simulink model "BatteryStoragePVPlantGFM"  (R2022b)
settings: Solver=FixedStepDiscrete  StartTime=0.0  StopTime=SimulationTime  RelTol=1e-3
PreLoadFcn:
  | run('BatteryStoragePVPlantGFMParameters')
undefined symbols (not defined in the file): Array, Base, battery, BatteryInverter, DiscIntNeverNeededParam, ee, Feeder, fRT, GFLBatteryController, GFMBatteryController, Grid, GridTransformer, Line, Load, Load2CB_final, Load2CB_initial, LVRT, maxSoC, maxVdc, minIrrad, minSoC, minVdc, Mpp, olTime, Panel, PVController, PVInverter, PVTransformer, Scenario, SM, SubTransmissionLine, Ts, VSMbase
libraries: ee_lib x51, nesl_utility x45, fl_lib x26, eeGeneralControl x18, simulink x12, eeTransforms x11, slpidlib x8, eePowerMeasurement x5, batteryecm_lib x2, eeTotalHarmonicDistorsion x2, spsLeadLagFilterLib x1, eeSmAC1C x1
(part 3 of 5)

== system BatteryStoragePVPlantGFM/BESS & PV PARK/PV Plant Controller /Voltage VAR Control & LVRT, FRT/Voltage Control ==
  In1 : Inport
  In2 : Inport  Port=2
  Constant2 : Constant  Value=0
  Gain : Gain  Gain=PVController.m_v
  Sum2 : Sum  Inputs=|+-
  Switch1 : Switch  Threshold=.9  SaturateOnIntegerOverflow=off  InputSameDT=off
  Out1 : Outport
  wires:
  Gain/1 -> Out1/1
  Sum2/1 -> Switch1/1
  Switch1/1 -> Gain/1
  In1/1 -> Sum2/2, Switch1/2
  Constant2/1 -> Switch1/3
  In2/1 -> Sum2/1

== system BatteryStoragePVPlantGFM/Conventional Source/Variant Subsystem/Frequency Controlled Source/Frequency Control ==
  Pref : Inport
  In Bus Element : Inport  Port=2  PortName=Grid  Element=Pe
  Discrete-Time Integrator : DiscreteIntegrator  IntegratorMethod=Integration: Backward Euler  InitialCondition=0.998  SampleTime=Ts  LimitOutput=on  UpperSaturationLimit=1.1  LowerSaturationLimit=0.9  ICPrevOutput=DiscIntNeverNeededParam  ICPrevScaledInput=DiscIntNeverNeededParam
  Gain2 : Gain  Gain=Grid.frequency
  Gain3 : Gain  Gain=1/Grid.H
  Gain4 : Gain  Gain=Grid.damping*2*pi*Grid.frequency
  Gain6 : Gain  Gain=1/Grid.governor_droop
  Sum : Sum  Inputs=|+-
  Sum1 : Sum  Inputs=-+-|
  Sum2 : Sum  Inputs=|+-
  Sum3 : Sum  Inputs=++|
  Unit Delay : UnitDelay  InitialCondition=1  SampleTime=Grid.sensor_time  HasFrameUpgradeWarning=on
  Unit Delay1 : UnitDelay  InitialCondition=1  SampleTime=Grid.sensor_time  HasFrameUpgradeWarning=on
  w_ref : Constant
  Frequency : Outport
  wires:
  Sum3/1 -> Sum1/2
  w_ref/1 -> Sum2/2, Sum/1
  Sum1/1 -> Gain3/1
  Gain3/1 -> Discrete-Time Integrator/1
  Gain6/1 -> Sum3/2
  Gain2/1 -> Frequency/1
  Sum2/1 -> Gain4/1
  Sum/1 -> Gain6/1
  Pref/1 -> Sum3/1
  Gain4/1 -> Sum1/3
  In Bus Element/1 -> Sum1/1
  Discrete-Time Integrator/1 -> Unit Delay1/1, Unit Delay/1, Gain2/1
  Unit Delay/1 -> Sum/2
  Unit Delay1/1 -> Sum2/1

== system BatteryStoragePVPlantGFM/Conventional Source/Variant Subsystem/Synchronous Machine/AVR and Exciter ==
  Constant{3,5..9} (6 alike) : Constant  Value=0
  Constant4 : Constant
  "E_FD Simulink-PS " : nesl_utility/Simulink-PS Converter  PhysicalDomain=network_engine_domain  SubClassName=ps_input  LeftPortType=input  RightPortType=output  PseudoPeriodic=off  Frequencies=[]  NoiseDistribution=none  NoiseParameters=[]  Unit=1  AffineConversion=off  FilteringAndDerivatives=provide  SimscapeFilterOrder=1  InputFilterTimeConstant=.001  UdotUserProvided=0
  I_FD PS-Simulink : nesl_utility/PS-Simulink Converter  PhysicalDomain=network_engine_domain  SubClassName=ps_output  LeftPortType=input  RightPortType=output  PseudoPeriodic=off  Frequencies=[]  VectorFormat=1-D array  Unit=1  AffineConversion=off
  SM AC1C : eeSmAC1C/SM AC1C  E_FD0=1  Ts=-1  R_C=0  X_C=0  T_R=0  K_A=600  T_A=0.01  T_B=0  T_C=0  K_F=0.35  T_F=0.5  V_Amax=14.5  V_Amin=-14.5  E_FEmax=6.03  E_FEmin=-5.43  oelInputLocation=Unused  uelInputLocation=Unused  sclInputLocation=Unused  K_E=1  T_E=0.08  K_C=0.2  K_D=0.38  E_1=4.18  S_E_E1=0.1  E_2=3.14  S_E_E2=0.03  V_FEmax=99  V_Emin=0
  Synchronous Machine Field Circuit (pu) : ee_lib/Electromechanical/Synchronous/Synchronous Machine Field Circuit  unit_option=ee.enum.unit.pu  SRated=SM.MVA V*A  FRated=60 Hz  fieldCircuitParameterization_option=2  baseEfd=92.95 V  baseIfd=1300 A  parameterization_option=2  Ladu=1.66  Rfd=0.0006  Xl=SM.lekage_reactance  Xd=SM.xd  Xdd=SM.xd_  Xddd=SM.xd_dash  d_option=ee.enum.circuit.open  Td0d=SM.Tdo_ s  Tdd=1.3260 s  Td0dd=SM.Tdo_dash s  Tddd=0.0230 s
      settings: InternalSimscapePortConfiguration="{\"Bottom\":[],\"Left\":[{\"id\":\"Efd_pu\",\"label\":\"Efd_pu\",\"type\":\"input\"},{\"id\":\"Ifd_pu\",\"label\":\"Ifd_pu\",\"type\":\"output\"}],\"Right\":[{\"id\":\"fd_p\",\"label\":\"fd+\",\"type\":\"foundation.electrical.electrical\"},{\"id\":\"fd_n\",\"label\":\"fd-\",\"type\":\"foundation.electrical.electrical\"}],\"Top\":[]}"
  Terminal Current Measurement : ee_lib/Electromechanical/Synchronous/Synchronous Machine Measurement  output_idx=15
      settings: InternalSimscapePortConfiguration="{\"Bottom\":[],\"Left\":[{\"id\":\"pu_input\",\"label\":\"pu\",\"type\":\"input\"}],\"Right\":[{\"id\":\"pu_output\",\"label\":\"o\",\"type\":\"output\"}],\"Top\":[]}"
  Terminal Current PS-Simulink : nesl_utility/PS-Simulink Converter  PhysicalDomain=network_engine_domain  SubClassName=ps_output  LeftPortType=input  RightPortType=output  PseudoPeriodic=off  Frequencies=[]  VectorFormat=1-D array  Unit=1  AffineConversion=off
  Terminal Voltage Measurement : ee_lib/Electromechanical/Synchronous/Synchronous Machine Measurement  output_idx=14
      settings: InternalSimscapePortConfiguration="{\"Bottom\":[],\"Left\":[{\"id\":\"pu_input\",\"label\":\"pu\",\"type\":\"input\"}],\"Right\":[{\"id\":\"pu_output\",\"label\":\"o\",\"type\":\"output\"}],\"Top\":[]}"
  Terminal Voltage PS-Simulink : nesl_utility/PS-Simulink Converter  PhysicalDomain=network_engine_domain  SubClassName=ps_output  LeftPortType=input  RightPortType=output  PseudoPeriodic=off  Frequencies=[]  VectorFormat=1-D array  Unit=1  AffineConversion=off
  Unit Delay : UnitDelay  InitialCondition=1.32943  SampleTime=-1  HasFrameUpgradeWarning=on
  pu : PMIOPort  Side=Left
  fd+ : PMIOPort  Port=2  Side=Right
  fd- : PMIOPort  Port=3  Side=Right
  wires:
  Terminal Current PS-Simulink/1 -> SM AC1C/4
  SM AC1C/1 -> "E_FD Simulink-PS "/1
  Unit Delay/1 -> SM AC1C/10
  Constant9/1 -> SM AC1C/9
  Constant8/1 -> SM AC1C/8
  Constant7/1 -> SM AC1C/7
  Constant6/1 -> SM AC1C/6
  Constant5/1 -> SM AC1C/5
  Constant4/1 -> SM AC1C/1
  Constant3/1 -> SM AC1C/2
  Terminal Voltage PS-Simulink/1 -> SM AC1C/3
  I_FD PS-Simulink/1 -> Unit Delay/1
  connections:
  Terminal Current Measurement/RConn1 -- Terminal Current PS-Simulink/LConn1
  Terminal Voltage Measurement/RConn1 -- Terminal Voltage PS-Simulink/LConn1
  pu/RConn1 -- Terminal Current Measurement/LConn1 -- Terminal Voltage Measurement/LConn1
  Synchronous Machine Field Circuit (pu)/RConn1 -- fd+/RConn1
  fd-/RConn1 -- Synchronous Machine Field Circuit (pu)/RConn2
  I_FD PS-Simulink/LConn1 -- Synchronous Machine Field Circuit (pu)/LConn2
  "E_FD Simulink-PS "/RConn1 -- Synchronous Machine Field Circuit (pu)/LConn1

== system BatteryStoragePVPlantGFM/Conventional Source/Variant Subsystem/Synchronous Machine/CB4 ==
  Circuit Breaker Step off3 : ee_lib/Switches & Breakers/Circuit Breaker (Three-Phase)  R_closed=0.001 Ohm  G_open=1e-4 1/Ohm  threshold=0.5 V  breaker_behavior=ee.enum.switches.breakerBehavior.zeroCrossingEnable
      settings: InternalSimscapePortConfiguration="{\"Bottom\":[],\"Left\":[{\"id\":\"vT\",\"label\":\"vT\",\"type\":\"input\"},{\"id\":\"N1\",\"label\":\"~1\",\"type\":\"foundation.electrical.three_phase\"}],\"Right\":[{\"id\":\"N2\",\"label\":\"~2\",\"type\":\"foundation.electrical.three_phase\"}],\"Top\":[]}"
  Simulink-PS Converter3 : nesl_utility/Simulink-PS Converter  PhysicalDomain=network_engine_domain  SubClassName=ps_input  LeftPortType=input  RightPortType=output  PseudoPeriodic=off  Frequencies=[]  NoiseDistribution=none  NoiseParameters=[]  Unit=1  AffineConversion=off  FilteringAndDerivatives=zero  SimscapeFilterOrder=1  InputFilterTimeConstant=0.001  UdotUserProvided=1
  Step off3 : Step  Time=0  After=0  SampleTime=Ts
  Conn2 : PMIOPort  Side=Left
  Conn1 : PMIOPort  Port=2  Side=Right
  wires:
  Step off3/1 -> Simulink-PS Converter3/1
  connections:
  Circuit Breaker Step off3/LConn2 -- Conn2/RConn1
  Circuit Breaker Step off3/LConn1 -- Simulink-PS Converter3/RConn1
  Circuit Breaker Step off3/RConn1 -- Conn1/RConn1

== system BatteryStoragePVPlantGFM/Conventional Source/Variant Subsystem/Synchronous Machine/Governor and Prime Mover  ==
  Governor : Subsystem
  Ideal Torque Source : fl_lib/Mechanical/Mechanical Sources/Ideal Torque Source
  Mechanical Rotational Reference : fl_lib/Mechanical/Rotational Elements/Mechanical Rotational Reference
  Non-reheat turbine : Subsystem
  PS-Simulink Converter : nesl_utility/PS-Simulink Converter  PhysicalDomain=network_engine_domain  SubClassName=ps_output  LeftPortType=input  RightPortType=output  PseudoPeriodic=off  Frequencies=[]  VectorFormat=1-D array  Unit=1  AffineConversion=off
  Rotor Velocity Measurement : ee_lib/Electromechanical/Synchronous/Synchronous Machine Measurement  output_idx=4
      settings: InternalSimscapePortConfiguration="{\"Bottom\":[],\"Left\":[{\"id\":\"pu_input\",\"label\":\"pu\",\"type\":\"input\"}],\"Right\":[{\"id\":\"pu_output\",\"label\":\"o\",\"type\":\"output\"}],\"Top\":[]}"
  Simulink-PS Converter : nesl_utility/Simulink-PS Converter  PhysicalDomain=network_engine_domain  SubClassName=ps_input  LeftPortType=input  RightPortType=output  PseudoPeriodic=off  Frequencies=[]  NoiseDistribution=none  NoiseParameters=[]  Unit=1  AffineConversion=off  FilteringAndDerivatives=zero  SimscapeFilterOrder=1  InputFilterTimeConstant=0.001  UdotUserProvided=1
  scale by base_torque : Gain  Gain=base_torque
  R : PMIOPort  Side=Right
  C : PMIOPort  Port=2  Side=Right
  pu : PMIOPort  Port=3  Side=Left
  wires:
  PS-Simulink Converter/1 -> Governor/1(pu_velocity)
  Governor/1(delta_y) -> Non-reheat turbine/1(delta_y)
  Non-reheat turbine/1(torque) -> scale by base_torque/1
  scale by base_torque/1 -> Simulink-PS Converter/1
  connections:
  C/RConn1 -- Ideal Torque Source/RConn2 -- Mechanical Rotational Reference/LConn1
  Ideal Torque Source/LConn1 -- R/RConn1
  pu/RConn1 -- Rotor Velocity Measurement/LConn1
  PS-Simulink Converter/LConn1 -- Rotor Velocity Measurement/RConn1
  Simulink-PS Converter/RConn1 -- Ideal Torque Source/RConn1

== system BatteryStoragePVPlantGFM/BESS & PV PARK/100 MWp PV Park/PV Inverter A1/PV & Inverter/Measurement1 ==
  u : Inport
  Lead-Lag (Discrete or Continuous) : eeGeneralControl/Lead-Lag (Discrete or Continuous)  T1=0  T2=PVController.t_sensor  B=inf  A=-inf  init_option=Inherited from block input  x0=0  Ts=Ts
      settings: LibrarySourceBlock=|
      | ee_sl_lib/General Control/Lead-Lag
      | (Discrete or Continuous)
  Out1 : Outport
  wires:
  Lead-Lag (Discrete or Continuous)/1 -> Out1/1
  u/1 -> Lead-Lag (Discrete or Continuous)/1

== system BatteryStoragePVPlantGFM/BESS & PV PARK/100 MWp PV Park/PV Inverter A1/PV & Inverter/Measurement2 ==
  u : Inport
  Lead-Lag (Discrete or Continuous) : eeGeneralControl/Lead-Lag (Discrete or Continuous)  T1=0  T2=PVController.t_sensor  B=inf  A=-inf  init_option=Inherited from block input  x0=0  Ts=Ts
      settings: LibrarySourceBlock=|
      | ee_sl_lib/General Control/Lead-Lag
      | (Discrete or Continuous)
  Out1 : Outport
  wires:
  Lead-Lag (Discrete or Continuous)/1 -> Out1/1
  u/1 -> Lead-Lag (Discrete or Continuous)/1

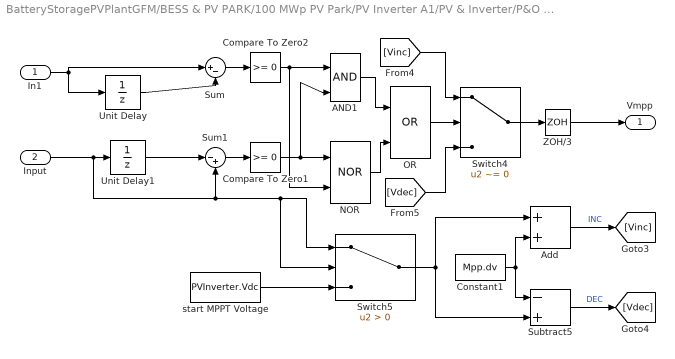
== system BatteryStoragePVPlantGFM/BESS & PV PARK/100 MWp PV Park/PV Inverter A1/PV & Inverter/P&O MPP ==
  In1 : Inport
  Input : Inport  Port=2
  AND1 : Logic  IconShape=distinctive  AllPortsSameDT=off  OutDataTypeStr=boolean
  Add : Sum
  Compare To Zero1 : simulink/Logic and Bit Operations/Compare To Zero  relop=>=  OutDataTypeStr=boolean
  Compare To Zero2 : simulink/Logic and Bit Operations/Compare To Zero  relop=>=  OutDataTypeStr=boolean
  Constant1 : Constant  Value=Mpp.dv
  NOR : Logic  Operator=NOR  IconShape=distinctive  AllPortsSameDT=off  OutDataTypeStr=boolean
  OR : Logic  Operator=OR  IconShape=distinctive  AllPortsSameDT=off  OutDataTypeStr=boolean
  Subtract5 : Sum  Inputs=-+
  Sum : Sum  Inputs=|+-
  Sum1 : Sum  Inputs=|-+
  Switch4 : Switch  Criteria=u2 ~= 0  SaturateOnIntegerOverflow=off  InputSameDT=off
  Switch5 : Switch  Criteria=u2 > Threshold  SaturateOnIntegerOverflow=off  InputSameDT=off
  Unit Delay : UnitDelay  InitialCondition=2.5e5  SampleTime=Mpp.ts  HasFrameUpgradeWarning=on
  Unit Delay1 : UnitDelay  InitialCondition=1*PVInverter.Vdc  SampleTime=Mpp.ts  HasFrameUpgradeWarning=on
  ZOH/3 : ZeroOrderHold  SampleTime=Mpp.td
  start MPPT Voltage : Constant  Value=PVInverter.Vdc  SampleTime=Ts
  Vmpp : Outport  VectorParamsAs1DForOutWhenUnconnected=off
  wires:
  OR/1 -> Switch4/2
  Compare To Zero1/1 -> NOR/1, AND1/2
  start MPPT Voltage/1 -> Switch5/3
  Compare To Zero2/1 -> NOR/2, AND1/1
  In1/1 -> Unit Delay/1, Sum/1
  Switch5/1 -> Add/1, Subtract5/2
  Constant1/1 -> Add/2, Subtract5/1
  Input/1 -> Switch5/2, Switch5/1, Sum1/2, Unit Delay1/1
  Unit Delay1/1 -> Sum1/1
  Add/1 -> [Vinc]  "INC"
  NOR/1 -> OR/2
  Subtract5/1 -> [Vdec]  "DEC"
  [Vdec] -> Switch4/3
  Switch4/1 -> ZOH/3/1
  Sum1/1 -> Compare To Zero1/1
  Sum/1 -> Compare To Zero2/1
  AND1/1 -> OR/1
  Unit Delay/1 -> Sum/2
  ZOH/3/1 -> Vmpp/1
  [Vinc] -> Switch4/1

== system BatteryStoragePVPlantGFM/BESS & PV PARK/100 MWp PV Park/PV Inverter A1/PV Controller/Current_controller ==
  id-ref : Inport
  ipvd : Inport  Port=2
  iqref : Inport  Port=3
  iq : Inport  Port=4
  Vd : Inport  Port=5
  Vq : Inport  Port=6
  Constant4 : Constant  Value=0
  Gain1 : Gain  Gain=2*1*pi*60*PVInverter.L/Base.z_base
  Gain2 : Gain  Gain=2*1*pi*60*PVInverter.L/Base.z_base
  Mux1 : Mux  Inputs=3
  PID Controller : slpidlib/PID Controller  Controller=PID  Form=Parallel  TimeDomain=Discrete-time  UseExternalTs=off  SampleTime=-1  IntegratorMethod=Forward Euler  FilterMethod=Forward Euler  ControllerParametersSource=internal  P=PVController.Kp_ic  I=PVController.Ki_ic  UseKiTs=off  D=PVController.Kd  N=100  UseFilter=on  TunerSelectOption=Transfer Function Based (PID Tuner App)  InitialConditionSource=internal  InitialConditionForIntegrator=0  InitialConditionForFilter=0  DifferentiatorICPrevScaledInput=0  ExternalReset=none  TrackingMode=off  Kt=1  LimitOutput=off  SatLimitsSource=internal  UpperSaturationLimit=inf  LowerSaturationLimit=-inf  LinearizeAsGain=on  AntiWindupMode=none  Kb=1  LimitIntegrator=off  UpperIntegratorSaturationLimit=inf  LowerIntegratorSaturationLimit=-inf  POutMin=[]  POutMax=[]  IOutMin=[]  IOutMax=[]  DOutMin=[]  DOutMax=[]  NOutMin=[]  NOutMax=[]  SumOutMin=[]  SumOutMax=[]  SaturationOutMin=[]  SaturationOutMax=[]  PParamMin=[]  PParamMax=[]  IParamMin=[]  IParamMax=[]  DParamMin=[]  DParamMax=[]  NParamMin=[]  NParamMax=[]  KbParamMin=[]  KbParamMax=[]  KtParamMin=[]  KtParamMax=[]  KbOutMin=[]  KbOutMax=[]  KtOutMin=[]  KtOutMax=[]  IntegratorOutMin=[]  IntegratorOutMax=[]  FilterOutMin=[]  FilterOutMax=[]  SumI1OutMin=[]  SumI1OutMax=[]  SumI2OutMin=[]  SumI2OutMax=[]  SumI3OutMin=[]  SumI3OutMax=[]  SumI4OutMin=[]  SumI4OutMax=[]  SumDOutMin=[]  SumDOutMax=[]  DifferentiatorOutMin=[]  DifferentiatorOutMax=[]  FilterDiffOutCoefMin=[]  FilterDiffOutCoefMax=[]  ReciprocalOutMin=[]  ReciprocalOutMax=[]  SumDenOutMin=[]  SumDenOutMax=[]  SumNumOutMin=[]  SumNumOutMax=[]  DivideOutMin=[]  DivideOutMax=[]  UdiffTsProdOutMin=[]  UdiffTsProdOutMax=[]  NTsProdOutMin=[]  NTsProdOutMax=[]  UintegralTsProdOutMin=[]  UintegralTsProdOutMax=[]  UngainTsProdOutMin=[]  UngainTsProdOutMax=[]  ClampingZeroOutDataTypeStr=Inherit: Inherit via back propagation  ClampingZeroOutMin=[]  ClampingZeroOutMax=[]  FilterDenConstantOutDataTypeStr=Inherit: Inherit via back propagation  FilterDenConstantOutMin=[]  FilterDenConstantOutMax=[]  PCopyOutDataTypeStr=Inherit: Inherit via back propagation  PCopyOutMin=[]  PCopyOutMax=[]  NCopyOutDataTypeStr=Inherit: Inherit via back propagation  NCopyOutMin=[]  NCopyOutMax=[]  IntegratorContinuousStateAttributes=''  IntegratorStateMustResolveToSignalObject=off  IntegratorRTWStateStorageClass=Auto  FilterContinuousStateAttributes=''  FilterStateMustResolveToSignalObject=off  FilterRTWStateStorageClass=Auto  ParallelPVariant=InternalParameters  IdealPVariant=Disabled  IVariant=InternalParameters  DVariant=InternalParameters  IntegratorVariant=Discrete  SatVariant=Disabled  AWVariant=Passthrough  PCopyVariant=Disabled  TRVariant=Disabled  FdbkBlocksVariant=Forward  IdealPFdbkVariant=Disabled  SatFdbkVariant=Disabled  DerivativeFilterVariant=ForwardEulerFilter  NVariant=InternalParameters  NCopyVariant=Disabled  FilterICVariant=InternalICsFilter  IntegratorICVariant=InternalICs  ExternalResetVariant=Disabled  TRSumVariant=Passthrough  SumFdbkVariant=Disabled  SumVariant=Sum_PID  TsampFilterVariant=InternalTs  TsampNgainVariant=Passthrough  TsampIntegralVariant=Passthrough  ExternalSaturationOutDataTypeStr=Inherit: Same as second input
  PID Controller1 : slpidlib/PID Controller  Controller=PID  Form=Parallel  TimeDomain=Discrete-time  UseExternalTs=off  SampleTime=-1  IntegratorMethod=Forward Euler  FilterMethod=Forward Euler  ControllerParametersSource=internal  P=PVController.Kp_ic  I=PVController.Ki_ic  UseKiTs=off  D=PVController.Kd  N=100  UseFilter=on  TunerSelectOption=Transfer Function Based (PID Tuner App)  InitialConditionSource=internal  InitialConditionForIntegrator=0  InitialConditionForFilter=0  DifferentiatorICPrevScaledInput=0  ExternalReset=none  TrackingMode=off  Kt=1  LimitOutput=off  SatLimitsSource=internal  UpperSaturationLimit=inf  LowerSaturationLimit=-inf  LinearizeAsGain=on  AntiWindupMode=none  Kb=1  LimitIntegrator=off  UpperIntegratorSaturationLimit=inf  LowerIntegratorSaturationLimit=-inf  POutMin=[]  POutMax=[]  IOutMin=[]  IOutMax=[]  DOutMin=[]  DOutMax=[]  NOutMin=[]  NOutMax=[]  SumOutMin=[]  SumOutMax=[]  SaturationOutMin=[]  SaturationOutMax=[]  PParamMin=[]  PParamMax=[]  IParamMin=[]  IParamMax=[]  DParamMin=[]  DParamMax=[]  NParamMin=[]  NParamMax=[]  KbParamMin=[]  KbParamMax=[]  KtParamMin=[]  KtParamMax=[]  KbOutMin=[]  KbOutMax=[]  KtOutMin=[]  KtOutMax=[]  IntegratorOutMin=[]  IntegratorOutMax=[]  FilterOutMin=[]  FilterOutMax=[]  SumI1OutMin=[]  SumI1OutMax=[]  SumI2OutMin=[]  SumI2OutMax=[]  SumI3OutMin=[]  SumI3OutMax=[]  SumI4OutMin=[]  SumI4OutMax=[]  SumDOutMin=[]  SumDOutMax=[]  DifferentiatorOutMin=[]  DifferentiatorOutMax=[]  FilterDiffOutCoefMin=[]  FilterDiffOutCoefMax=[]  ReciprocalOutMin=[]  ReciprocalOutMax=[]  SumDenOutMin=[]  SumDenOutMax=[]  SumNumOutMin=[]  SumNumOutMax=[]  DivideOutMin=[]  DivideOutMax=[]  UdiffTsProdOutMin=[]  UdiffTsProdOutMax=[]  NTsProdOutMin=[]  NTsProdOutMax=[]  UintegralTsProdOutMin=[]  UintegralTsProdOutMax=[]  UngainTsProdOutMin=[]  UngainTsProdOutMax=[]  ClampingZeroOutDataTypeStr=Inherit: Inherit via back propagation  ClampingZeroOutMin=[]  ClampingZeroOutMax=[]  FilterDenConstantOutDataTypeStr=Inherit: Inherit via back propagation  FilterDenConstantOutMin=[]  FilterDenConstantOutMax=[]  PCopyOutDataTypeStr=Inherit: Inherit via back propagation  PCopyOutMin=[]  PCopyOutMax=[]  NCopyOutDataTypeStr=Inherit: Inherit via back propagation  NCopyOutMin=[]  NCopyOutMax=[]  IntegratorContinuousStateAttributes=''  IntegratorStateMustResolveToSignalObject=off  IntegratorRTWStateStorageClass=Auto  FilterContinuousStateAttributes=''  FilterStateMustResolveToSignalObject=off  FilterRTWStateStorageClass=Auto  ParallelPVariant=InternalParameters  IdealPVariant=Disabled  IVariant=InternalParameters  DVariant=InternalParameters  IntegratorVariant=Discrete  SatVariant=Disabled  AWVariant=Passthrough  PCopyVariant=Disabled  TRVariant=Disabled  FdbkBlocksVariant=Forward  IdealPFdbkVariant=Disabled  SatFdbkVariant=Disabled  DerivativeFilterVariant=ForwardEulerFilter  NVariant=InternalParameters  NCopyVariant=Disabled  FilterICVariant=InternalICsFilter  IntegratorICVariant=InternalICs  ExternalResetVariant=Disabled  TRSumVariant=Passthrough  SumFdbkVariant=Disabled  SumVariant=Sum_PID  TsampFilterVariant=InternalTs  TsampNgainVariant=Passthrough  TsampIntegralVariant=Passthrough  ExternalSaturationOutDataTypeStr=Inherit: Same as second input
  Sum1 : Sum  Inputs=|+-
  Sum3 : Sum  Inputs=|++-
  Sum4 : Sum  Inputs=|+++
  Sum5 : Sum  Inputs=|+-
  Refrence_mdq0 : Outport
  wires:
  PID Controller/1 -> Sum3/2
  Sum3/1 -> Mux1/1, [Ed]
  Gain2/1 -> Sum3/3
  ipvd/1 -> Gain1/1, Sum1/2
  id-ref/1 -> Sum1/1
  Gain1/1 -> Sum4/3
  Vq/1 -> Sum4/2
  iq/1 -> Gain2/1, Sum5/2
  Sum1/1 -> PID Controller/1
  Vd/1 -> Sum3/1
  Constant4/1 -> Mux1/3
  Sum5/1 -> PID Controller1/1
  iqref/1 -> Sum5/1
  PID Controller1/1 -> Sum4/1
  Sum4/1 -> Mux1/2, [Eq]
  Mux1/1 -> Refrence_mdq0/1  "m_dqo"

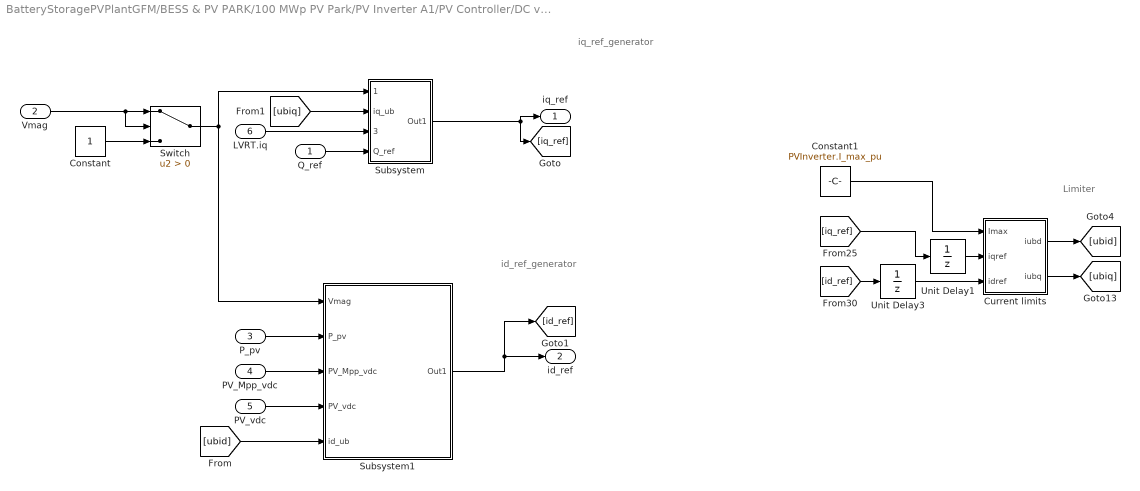
== system BatteryStoragePVPlantGFM/BESS & PV PARK/100 MWp PV Park/PV Inverter A1/PV Controller/DC voltage controller & current reference ==
  note: Limiter
  note: iq_ref_generator
  note: id_ref_generator
  Q_ref : Inport
  Vmag : Inport  Port=2
  P_pv : Inport  Port=3
  PV_Mpp_vdc : Inport  Port=4
  PV_vdc : Inport  Port=5
  LVRT.iq : Inport  Port=6
  Constant : Constant
  Constant1 : Constant  Value=PVInverter.I_max_pu
  Current limits : Subsystem
  Subsystem : Subsystem
  Subsystem1 : Subsystem
  Switch : Switch  Criteria=u2 > Threshold  SaturateOnIntegerOverflow=off  InputSameDT=off
  Unit Delay1 : UnitDelay  SampleTime=Ts  HasFrameUpgradeWarning=on
  Unit Delay3 : UnitDelay  SampleTime=Ts  HasFrameUpgradeWarning=on
  iq_ref : Outport
  id_ref : Outport  Port=2
  wires:
  Vmag/1 -> Switch/2, Switch/1
  [iq_ref] -> Unit Delay1/1
  Current limits/2(iubq) -> [ubiq]
  Current limits/1(iubd) -> [ubid]
  Constant1/1 -> Current limits/1(Imax)
  Unit Delay1/1 -> Current limits/2(iqref)
  [id_ref] -> Unit Delay3/1
  Unit Delay3/1 -> Current limits/3(idref)
  Q_ref/1 -> Subsystem/4(Q_ref)
  Subsystem1/1(Out1) -> [id_ref], id_ref/1
  P_pv/1 -> Subsystem1/2(P_pv)
  PV_Mpp_vdc/1 -> Subsystem1/3(PV_Mpp_vdc)
  PV_vdc/1 -> Subsystem1/4(PV_vdc)
  Subsystem/1(Out1) -> [iq_ref], iq_ref/1
  [ubid] -> Subsystem1/5(id_ub)
  [ubiq] -> Subsystem/2(iq_ub)
  LVRT.iq/1 -> Subsystem/3(LVRT.iq)
  Switch/1 -> Subsystem/1(V_mag), Subsystem1/1(Vmag)
  Constant/1 -> Switch/3

== system BatteryStoragePVPlantGFM/BESS & PV PARK/100 MWp PV Park/PV Inverter A2/PV & Inverter/Measurement1 ==
  u : Inport
  Lead-Lag (Discrete or Continuous) : eeGeneralControl/Lead-Lag (Discrete or Continuous)  T1=0  T2=PVController.t_sensor  B=inf  A=-inf  init_option=Inherited from block input  x0=0  Ts=Ts
      settings: LibrarySourceBlock=|
      | ee_sl_lib/General Control/Lead-Lag
      | (Discrete or Continuous)
  Out1 : Outport
  wires:
  Lead-Lag (Discrete or Continuous)/1 -> Out1/1
  u/1 -> Lead-Lag (Discrete or Continuous)/1

== system BatteryStoragePVPlantGFM/BESS & PV PARK/100 MWp PV Park/PV Inverter A2/PV & Inverter/Measurement2 ==
  u : Inport
  Lead-Lag (Discrete or Continuous) : eeGeneralControl/Lead-Lag (Discrete or Continuous)  T1=0  T2=PVController.t_sensor  B=inf  A=-inf  init_option=Inherited from block input  x0=0  Ts=Ts
      settings: LibrarySourceBlock=|
      | ee_sl_lib/General Control/Lead-Lag
      | (Discrete or Continuous)
  Out1 : Outport
  wires:
  Lead-Lag (Discrete or Continuous)/1 -> Out1/1
  u/1 -> Lead-Lag (Discrete or Continuous)/1

== system BatteryStoragePVPlantGFM/BESS & PV PARK/100 MWp PV Park/PV Inverter A2/PV & Inverter/P&O MPP ==
  In1 : Inport
  Input : Inport  Port=2
  AND1 : Logic  IconShape=distinctive  AllPortsSameDT=off  OutDataTypeStr=boolean
  Add : Sum
  Compare To Zero1 : simulink/Logic and Bit Operations/Compare To Zero  relop=>=  OutDataTypeStr=boolean
  Compare To Zero2 : simulink/Logic and Bit Operations/Compare To Zero  relop=>=  OutDataTypeStr=boolean
  Constant1 : Constant  Value=Mpp.dv
  NOR : Logic  Operator=NOR  IconShape=distinctive  AllPortsSameDT=off  OutDataTypeStr=boolean
  OR : Logic  Operator=OR  IconShape=distinctive  AllPortsSameDT=off  OutDataTypeStr=boolean
  Subtract5 : Sum  Inputs=-+
  Sum : Sum  Inputs=|+-
  Sum1 : Sum  Inputs=|-+
  Switch4 : Switch  Criteria=u2 ~= 0  SaturateOnIntegerOverflow=off  InputSameDT=off
  Switch5 : Switch  Criteria=u2 > Threshold  SaturateOnIntegerOverflow=off  InputSameDT=off
  Unit Delay : UnitDelay  InitialCondition=2.5e5  SampleTime=Mpp.ts  HasFrameUpgradeWarning=on
  Unit Delay1 : UnitDelay  InitialCondition=1*PVInverter.Vdc  SampleTime=Mpp.ts  HasFrameUpgradeWarning=on
  ZOH/3 : ZeroOrderHold  SampleTime=Mpp.td
  start MPPT Voltage : Constant  Value=PVInverter.Vdc  SampleTime=Ts
  Vmpp : Outport  VectorParamsAs1DForOutWhenUnconnected=off
  wires:
  OR/1 -> Switch4/2
  Compare To Zero1/1 -> NOR/1, AND1/2
  start MPPT Voltage/1 -> Switch5/3
  Compare To Zero2/1 -> NOR/2, AND1/1
  In1/1 -> Unit Delay/1, Sum/1
  Switch5/1 -> Add/1, Subtract5/2
  Constant1/1 -> Add/2, Subtract5/1
  Input/1 -> Switch5/2, Switch5/1, Sum1/2, Unit Delay1/1
  Unit Delay1/1 -> Sum1/1
  Add/1 -> [Vinc]  "INC"
  NOR/1 -> OR/2
  Subtract5/1 -> [Vdec]  "DEC"
  [Vdec] -> Switch4/3
  Switch4/1 -> ZOH/3/1
  Sum1/1 -> Compare To Zero1/1
  Sum/1 -> Compare To Zero2/1
  AND1/1 -> OR/1
  Unit Delay/1 -> Sum/2
  ZOH/3/1 -> Vmpp/1
  [Vinc] -> Switch4/1

== system BatteryStoragePVPlantGFM/BESS & PV PARK/100 MWp PV Park/PV Inverter A2/PV Controller/Current_controller ==
  id-ref : Inport
  ipvd : Inport  Port=2
  iqref : Inport  Port=3
  iq : Inport  Port=4
  Vd : Inport  Port=5
  Vq : Inport  Port=6
  Constant4 : Constant  Value=0
  Gain1 : Gain  Gain=2*1*pi*60*PVInverter.L/Base.z_base
  Gain2 : Gain  Gain=2*1*pi*60*PVInverter.L/Base.z_base
  Mux1 : Mux  Inputs=3
  PID Controller : slpidlib/PID Controller  Controller=PID  Form=Parallel  TimeDomain=Discrete-time  UseExternalTs=off  SampleTime=-1  IntegratorMethod=Forward Euler  FilterMethod=Forward Euler  ControllerParametersSource=internal  P=PVController.Kp_ic  I=PVController.Ki_ic  UseKiTs=off  D=PVController.Kd  N=100  UseFilter=on  TunerSelectOption=Transfer Function Based (PID Tuner App)  InitialConditionSource=internal  InitialConditionForIntegrator=0  InitialConditionForFilter=0  DifferentiatorICPrevScaledInput=0  ExternalReset=none  TrackingMode=off  Kt=1  LimitOutput=off  SatLimitsSource=internal  UpperSaturationLimit=inf  LowerSaturationLimit=-inf  LinearizeAsGain=on  AntiWindupMode=none  Kb=1  LimitIntegrator=off  UpperIntegratorSaturationLimit=inf  LowerIntegratorSaturationLimit=-inf  POutMin=[]  POutMax=[]  IOutMin=[]  IOutMax=[]  DOutMin=[]  DOutMax=[]  NOutMin=[]  NOutMax=[]  SumOutMin=[]  SumOutMax=[]  SaturationOutMin=[]  SaturationOutMax=[]  PParamMin=[]  PParamMax=[]  IParamMin=[]  IParamMax=[]  DParamMin=[]  DParamMax=[]  NParamMin=[]  NParamMax=[]  KbParamMin=[]  KbParamMax=[]  KtParamMin=[]  KtParamMax=[]  KbOutMin=[]  KbOutMax=[]  KtOutMin=[]  KtOutMax=[]  IntegratorOutMin=[]  IntegratorOutMax=[]  FilterOutMin=[]  FilterOutMax=[]  SumI1OutMin=[]  SumI1OutMax=[]  SumI2OutMin=[]  SumI2OutMax=[]  SumI3OutMin=[]  SumI3OutMax=[]  SumI4OutMin=[]  SumI4OutMax=[]  SumDOutMin=[]  SumDOutMax=[]  DifferentiatorOutMin=[]  DifferentiatorOutMax=[]  FilterDiffOutCoefMin=[]  FilterDiffOutCoefMax=[]  ReciprocalOutMin=[]  ReciprocalOutMax=[]  SumDenOutMin=[]  SumDenOutMax=[]  SumNumOutMin=[]  SumNumOutMax=[]  DivideOutMin=[]  DivideOutMax=[]  UdiffTsProdOutMin=[]  UdiffTsProdOutMax=[]  NTsProdOutMin=[]  NTsProdOutMax=[]  UintegralTsProdOutMin=[]  UintegralTsProdOutMax=[]  UngainTsProdOutMin=[]  UngainTsProdOutMax=[]  ClampingZeroOutDataTypeStr=Inherit: Inherit via back propagation  ClampingZeroOutMin=[]  ClampingZeroOutMax=[]  FilterDenConstantOutDataTypeStr=Inherit: Inherit via back propagation  FilterDenConstantOutMin=[]  FilterDenConstantOutMax=[]  PCopyOutDataTypeStr=Inherit: Inherit via back propagation  PCopyOutMin=[]  PCopyOutMax=[]  NCopyOutDataTypeStr=Inherit: Inherit via back propagation  NCopyOutMin=[]  NCopyOutMax=[]  IntegratorContinuousStateAttributes=''  IntegratorStateMustResolveToSignalObject=off  IntegratorRTWStateStorageClass=Auto  FilterContinuousStateAttributes=''  FilterStateMustResolveToSignalObject=off  FilterRTWStateStorageClass=Auto  ParallelPVariant=InternalParameters  IdealPVariant=Disabled  IVariant=InternalParameters  DVariant=InternalParameters  IntegratorVariant=Discrete  SatVariant=Disabled  AWVariant=Passthrough  PCopyVariant=Disabled  TRVariant=Disabled  FdbkBlocksVariant=Forward  IdealPFdbkVariant=Disabled  SatFdbkVariant=Disabled  DerivativeFilterVariant=ForwardEulerFilter  NVariant=InternalParameters  NCopyVariant=Disabled  FilterICVariant=InternalICsFilter  IntegratorICVariant=InternalICs  ExternalResetVariant=Disabled  TRSumVariant=Passthrough  SumFdbkVariant=Disabled  SumVariant=Sum_PID  TsampFilterVariant=InternalTs  TsampNgainVariant=Passthrough  TsampIntegralVariant=Passthrough  ExternalSaturationOutDataTypeStr=Inherit: Same as second input
  PID Controller1 : slpidlib/PID Controller  Controller=PID  Form=Parallel  TimeDomain=Discrete-time  UseExternalTs=off  SampleTime=-1  IntegratorMethod=Forward Euler  FilterMethod=Forward Euler  ControllerParametersSource=internal  P=PVController.Kp_ic  I=PVController.Ki_ic  UseKiTs=off  D=PVController.Kd  N=100  UseFilter=on  TunerSelectOption=Transfer Function Based (PID Tuner App)  InitialConditionSource=internal  InitialConditionForIntegrator=0  InitialConditionForFilter=0  DifferentiatorICPrevScaledInput=0  ExternalReset=none  TrackingMode=off  Kt=1  LimitOutput=off  SatLimitsSource=internal  UpperSaturationLimit=inf  LowerSaturationLimit=-inf  LinearizeAsGain=on  AntiWindupMode=none  Kb=1  LimitIntegrator=off  UpperIntegratorSaturationLimit=inf  LowerIntegratorSaturationLimit=-inf  POutMin=[]  POutMax=[]  IOutMin=[]  IOutMax=[]  DOutMin=[]  DOutMax=[]  NOutMin=[]  NOutMax=[]  SumOutMin=[]  SumOutMax=[]  SaturationOutMin=[]  SaturationOutMax=[]  PParamMin=[]  PParamMax=[]  IParamMin=[]  IParamMax=[]  DParamMin=[]  DParamMax=[]  NParamMin=[]  NParamMax=[]  KbParamMin=[]  KbParamMax=[]  KtParamMin=[]  KtParamMax=[]  KbOutMin=[]  KbOutMax=[]  KtOutMin=[]  KtOutMax=[]  IntegratorOutMin=[]  IntegratorOutMax=[]  FilterOutMin=[]  FilterOutMax=[]  SumI1OutMin=[]  SumI1OutMax=[]  SumI2OutMin=[]  SumI2OutMax=[]  SumI3OutMin=[]  SumI3OutMax=[]  SumI4OutMin=[]  SumI4OutMax=[]  SumDOutMin=[]  SumDOutMax=[]  DifferentiatorOutMin=[]  DifferentiatorOutMax=[]  FilterDiffOutCoefMin=[]  FilterDiffOutCoefMax=[]  ReciprocalOutMin=[]  ReciprocalOutMax=[]  SumDenOutMin=[]  SumDenOutMax=[]  SumNumOutMin=[]  SumNumOutMax=[]  DivideOutMin=[]  DivideOutMax=[]  UdiffTsProdOutMin=[]  UdiffTsProdOutMax=[]  NTsProdOutMin=[]  NTsProdOutMax=[]  UintegralTsProdOutMin=[]  UintegralTsProdOutMax=[]  UngainTsProdOutMin=[]  UngainTsProdOutMax=[]  ClampingZeroOutDataTypeStr=Inherit: Inherit via back propagation  ClampingZeroOutMin=[]  ClampingZeroOutMax=[]  FilterDenConstantOutDataTypeStr=Inherit: Inherit via back propagation  FilterDenConstantOutMin=[]  FilterDenConstantOutMax=[]  PCopyOutDataTypeStr=Inherit: Inherit via back propagation  PCopyOutMin=[]  PCopyOutMax=[]  NCopyOutDataTypeStr=Inherit: Inherit via back propagation  NCopyOutMin=[]  NCopyOutMax=[]  IntegratorContinuousStateAttributes=''  IntegratorStateMustResolveToSignalObject=off  IntegratorRTWStateStorageClass=Auto  FilterContinuousStateAttributes=''  FilterStateMustResolveToSignalObject=off  FilterRTWStateStorageClass=Auto  ParallelPVariant=InternalParameters  IdealPVariant=Disabled  IVariant=InternalParameters  DVariant=InternalParameters  IntegratorVariant=Discrete  SatVariant=Disabled  AWVariant=Passthrough  PCopyVariant=Disabled  TRVariant=Disabled  FdbkBlocksVariant=Forward  IdealPFdbkVariant=Disabled  SatFdbkVariant=Disabled  DerivativeFilterVariant=ForwardEulerFilter  NVariant=InternalParameters  NCopyVariant=Disabled  FilterICVariant=InternalICsFilter  IntegratorICVariant=InternalICs  ExternalResetVariant=Disabled  TRSumVariant=Passthrough  SumFdbkVariant=Disabled  SumVariant=Sum_PID  TsampFilterVariant=InternalTs  TsampNgainVariant=Passthrough  TsampIntegralVariant=Passthrough  ExternalSaturationOutDataTypeStr=Inherit: Same as second input
  Sum1 : Sum  Inputs=|+-
  Sum3 : Sum  Inputs=|++-
  Sum4 : Sum  Inputs=|+++
  Sum5 : Sum  Inputs=|+-
  Refrence_mdq0 : Outport
  wires:
  PID Controller/1 -> Sum3/2
  Sum3/1 -> Mux1/1, [Ed]
  Gain2/1 -> Sum3/3
  ipvd/1 -> Gain1/1, Sum1/2
  id-ref/1 -> Sum1/1
  Gain1/1 -> Sum4/3
  Vq/1 -> Sum4/2
  iq/1 -> Gain2/1, Sum5/2
  Sum1/1 -> PID Controller/1
  Vd/1 -> Sum3/1
  Constant4/1 -> Mux1/3
  Sum5/1 -> PID Controller1/1
  iqref/1 -> Sum5/1
  PID Controller1/1 -> Sum4/1
  Sum4/1 -> Mux1/2, [Eq]
  Mux1/1 -> Refrence_mdq0/1  "m_dqo"

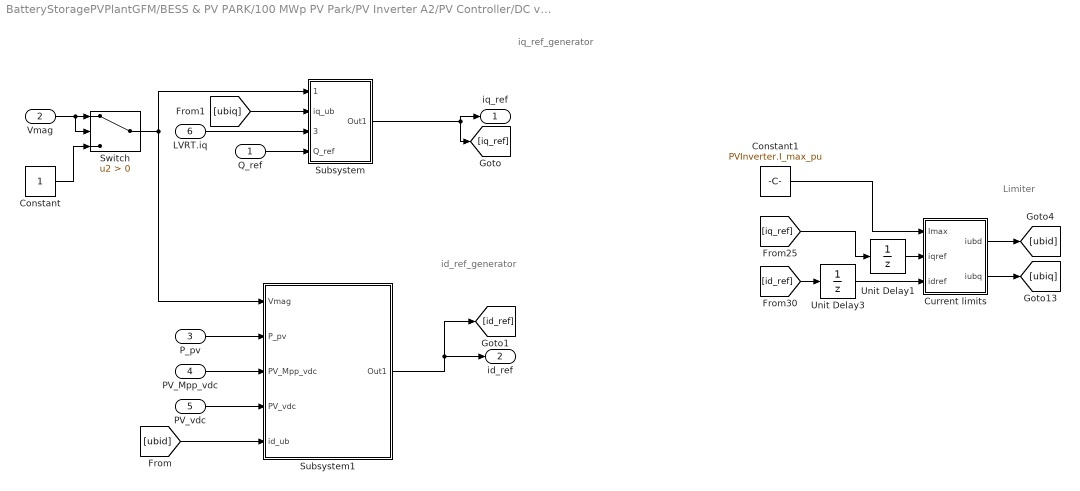
== system BatteryStoragePVPlantGFM/BESS & PV PARK/100 MWp PV Park/PV Inverter A2/PV Controller/DC voltage controller & current reference ==
  note: Limiter
  note: iq_ref_generator
  note: id_ref_generator
  Q_ref : Inport
  Vmag : Inport  Port=2
  P_pv : Inport  Port=3
  PV_Mpp_vdc : Inport  Port=4
  PV_vdc : Inport  Port=5
  LVRT.iq : Inport  Port=6
  Constant : Constant
  Constant1 : Constant  Value=PVInverter.I_max_pu
  Current limits : Subsystem
  Subsystem : Subsystem
  Subsystem1 : Subsystem
  Switch : Switch  Criteria=u2 > Threshold  SaturateOnIntegerOverflow=off  InputSameDT=off
  Unit Delay1 : UnitDelay  SampleTime=Ts  HasFrameUpgradeWarning=on
  Unit Delay3 : UnitDelay  SampleTime=Ts  HasFrameUpgradeWarning=on
  iq_ref : Outport
  id_ref : Outport  Port=2
  wires:
  [iq_ref] -> Unit Delay1/1
  Current limits/2(iubq) -> [ubiq]
  Current limits/1(iubd) -> [ubid]
  Constant1/1 -> Current limits/1(Imax)
  Unit Delay1/1 -> Current limits/2(iqref)
  [id_ref] -> Unit Delay3/1
  Unit Delay3/1 -> Current limits/3(idref)
  Q_ref/1 -> Subsystem/4(Q_ref)
  Subsystem1/1(Out1) -> [id_ref], id_ref/1
  P_pv/1 -> Subsystem1/2(P_pv)
  PV_Mpp_vdc/1 -> Subsystem1/3(PV_Mpp_vdc)
  PV_vdc/1 -> Subsystem1/4(PV_vdc)
  Subsystem/1(Out1) -> [iq_ref], iq_ref/1
  [ubid] -> Subsystem1/5(id_ub)
  [ubiq] -> Subsystem/2(iq_ub)
  LVRT.iq/1 -> Subsystem/3(LVRT.iq)
  Vmag/1 -> Switch/2, Switch/1
  Switch/1 -> Subsystem/1(V_mag), Subsystem1/1(Vmag)
  Constant/1 -> Switch/3

== system BatteryStoragePVPlantGFM/BESS & PV PARK/60 MWhr Battery Energy Storage/Variant Subsystem/Grid Following Support/Battery Inverter ==
  In Bus Element : Inport  PortName=Vbus
  In Bus Element1 : Inport  Port=2  PortName=ipv2
  LVRT_iq : Inport  Port=3
  GFL Battery Controller : Subsystem
  Inverter : Subsystem
  abc : PMIOPort  Side=Right
  wires:
  In Bus Element1/1 -> GFL Battery Controller/2(ipv2)
  GFL Battery Controller/1(m_abc) -> [m]
  In Bus Element/1 -> GFL Battery Controller/1(Vbus)
  LVRT_iq/1 -> GFL Battery Controller/3(LVRT_iq)
  [m] -> Inverter/1(m_abc)
  connections:
  abc/RConn1 -- Inverter/RConn1

== system BatteryStoragePVPlantGFM/BESS & PV PARK/60 MWhr Battery Energy Storage/Variant Subsystem/Grid Following Support/Measurement5 ==
  In1 : Inport
  u : Inport  Port=2
  Gain : Gain  Gain=sqrt((2/3))*Base.KV_base_new
  Gain1 : Gain  Gain=sqrt((1/3))*(Base.MVA_base_new/Base.KV_base_new)
  Lead-Lag (Discrete or Continuous) : eeGeneralControl/Lead-Lag (Discrete or Continuous)  T1=0  T2=PVController.t_sensor  B=inf  A=-inf  init_option=Inherited from block input  x0=0  Ts=Ts
      settings: LibrarySourceBlock=|
      | ee_sl_lib/General Control/Lead-Lag
      | (Discrete or Continuous)
  Lead-Lag (Discrete or Continuous)1 : eeGeneralControl/Lead-Lag (Discrete or Continuous)  T1=0  T2=PVController.t_sensor  B=inf  A=-inf  init_option=Inherited from block input  x0=0  Ts=Ts
      settings: LibrarySourceBlock=|
      | ee_sl_lib/General Control/Lead-Lag
      | (Discrete or Continuous)
  Out Bus Element : Outport  PortName=ipv1  Element=1
  Out Bus Element1 : Outport  Port=2  PortName=Bat  Element=Vabc_bat
  Out Bus Element2 : Outport  Port=2  PortName=Bat  Element=Iabc_bat
  wires:
  u/1 -> Lead-Lag (Discrete or Continuous)1/1
  Lead-Lag (Discrete or Continuous)1/1 -> Gain1/1, Out Bus Element/1
  In1/1 -> Lead-Lag (Discrete or Continuous)/1
  Lead-Lag (Discrete or Continuous)/1 -> Gain/1
  Gain/1 -> Out Bus Element1/1
  Gain1/1 -> Out Bus Element2/1

== system BatteryStoragePVPlantGFM/BESS & PV PARK/60 MWhr Battery Energy Storage/Variant Subsystem/Grid Forming VSM/Battery Inverter B1 ==
  In Bus Element : Inport  PortName=Bat
  Inverter : Subsystem
  controller : Subsystem
  abc : PMIOPort  Side=Right
  wires:
  [m] -> Inverter/1(reference)
  controller/1(mabc) -> [m]
  In Bus Element/1 -> controller/1(Bat)
  connections:
  abc/RConn1 -- Inverter/RConn1

== system BatteryStoragePVPlantGFM/BESS & PV PARK/60 MWhr Battery Energy Storage/Variant Subsystem/Grid Forming VSM/Filter & Sensor ==
  Current Sensor (Three-Phase) : ee_lib/Sensors & Transducers/Current Sensor (Three-Phase)
  Electrical Reference1 : fl_lib/Electrical/Electrical Elements/Electrical Reference
  Grounded Neutral (Three-Phase) : ee_lib/Connectors & References/Grounded Neutral (Three-Phase)
  Low-Pass Filter (Discrete or Continuous) : eeGeneralControl/Low-Pass Filter (Discrete or Continuous)  K=1  T=PVController.t_sensor  B=inf  A=-inf  init_option=Inherited from block input  x0=0  Ts=Ts
  Low-Pass Filter (Discrete or Continuous)1 : eeGeneralControl/Low-Pass Filter (Discrete or Continuous)  K=1  T=PVController.t_sensor  B=inf  A=-inf  init_option=Inherited from block input  x0=0  Ts=Ts
  Neutral Port (Three-Phase) : ee_lib/Connectors & References/Neutral Port (Three-Phase)  G_parasitic=1e-12 1/Ohm
      settings: InternalSimscapePortConfiguration="{\"Bottom\":[],\"Left\":[{\"id\":\"N\",\"label\":\"~\",\"type\":\"foundation.electrical.three_phase\"}],\"Right\":[{\"id\":\"n\",\"label\":\"n\",\"type\":\"foundation.electrical.electrical\"}],\"Top\":[]}"
  PS-Simulink Converter : nesl_utility/PS-Simulink Converter  PhysicalDomain=network_engine_domain  SubClassName=ps_output  LeftPortType=input  RightPortType=output  PseudoPeriodic=off  Frequencies=[]  VectorFormat=inherit  Unit=inherit  AffineConversion=off
  PS-Simulink Converter1 : nesl_utility/PS-Simulink Converter  PhysicalDomain=network_engine_domain  SubClassName=ps_output  LeftPortType=input  RightPortType=output  PseudoPeriodic=off  Frequencies=[]  VectorFormat=inherit  Unit=inherit  AffineConversion=off
  Phase Voltage Sensor (Three-Phase) : ee_lib/Sensors & Transducers/Phase Voltage Sensor (Three-Phase)
  RLC (Three-Phase) : ee_lib/Passive/RLC Assemblies/RLC (Three-Phase)  component_structure=ee.enum.rlc.structure.L  R=BatteryInverter.lineResistance Ohm  L=GFMBatteryController.L_bat H  C=1e-6 F  R_parasitic=0 Ohm  G_parasitic=0 1/Ohm  IL_specify=off  IL_priority=High  IL=[0, 0, 0] A  IL_nominal_specify=off  IL_nominal_unit=A  IL_nominal_value=1  VC_specify=off  VC_priority=High  VC=[0, 0, 0] V  VC_nominal_specify=off  VC_nominal_unit=V  VC_nominal_value=1
      settings: InternalSimscapePortConfiguration="{\"Bottom\":[],\"Left\":[{\"id\":\"N1\",\"label\":\"~1\",\"type\":\"foundation.electrical.three_phase\"}],\"Right\":[{\"id\":\"N2\",\"label\":\"~2\",\"type\":\"foundation.electrical.three_phase\"}],\"Top\":[]}"
  RLC (Three-Phase)1 : ee_lib/Passive/RLC Assemblies/RLC (Three-Phase)  component_structure=ee.enum.rlc.structure.C  R=BatteryInverter.lineResistance Ohm  L=BatteryInverter.L H  C=GFMBatteryController.C_bat F  R_parasitic=0 Ohm  G_parasitic=0 1/Ohm  IL_specify=off  IL_priority=High  IL=[0, 0, 0] A  IL_nominal_specify=off  IL_nominal_unit=A  IL_nominal_value=1  VC_specify=off  VC_priority=High  VC=[0, 0, 0] V  VC_nominal_specify=off  VC_nominal_unit=V  VC_nominal_value=1
      settings: InternalSimscapePortConfiguration="{\"Bottom\":[],\"Left\":[{\"id\":\"N1\",\"label\":\"~1\",\"type\":\"foundation.electrical.three_phase\"}],\"Right\":[{\"id\":\"N2\",\"label\":\"~2\",\"type\":\"foundation.electrical.three_phase\"}],\"Top\":[]}"
  Inabc : PMIOPort  Side=Left
  Opabc : PMIOPort  Port=2  Side=Right
  Out Bus Element : Outport  PortName=Bat  Element=Iabc_bat
  Out Bus Element1 : Outport  PortName=Bat  Element=Vabc_bat
  wires:
  PS-Simulink Converter/1 -> Low-Pass Filter (Discrete or Continuous)/1
  Low-Pass Filter (Discrete or Continuous)/1 -> Out Bus Element/1
  PS-Simulink Converter1/1 -> Low-Pass Filter (Discrete or Continuous)1/1
  Low-Pass Filter (Discrete or Continuous)1/1 -> Out Bus Element1/1
  connections:
  Electrical Reference1/LConn1 -- Neutral Port (Three-Phase)/RConn1
  PS-Simulink Converter1/LConn1 -- Phase Voltage Sensor (Three-Phase)/RConn1
  RLC (Three-Phase)1/LConn1 -- Current Sensor (Three-Phase)/LConn1 -- RLC (Three-Phase)/RConn1
  Neutral Port (Three-Phase)/LConn1 -- Phase Voltage Sensor (Three-Phase)/RConn2
  PS-Simulink Converter/LConn1 -- Current Sensor (Three-Phase)/RConn1
  Grounded Neutral (Three-Phase)/LConn1 -- RLC (Three-Phase)1/RConn1
  Inabc/RConn1 -- RLC (Three-Phase)/LConn1
  Phase Voltage Sensor (Three-Phase)/LConn1 -- Current Sensor (Three-Phase)/RConn2 -- Opabc/RConn1

== system BatteryStoragePVPlantGFM/BESS & PV PARK/PV Plant Controller /Voltage VAR Control & LVRT, FRT/Frequency RideThrough/Avoid Operation ==
  f_in : Inport
  Constant : Constant  Value=Grid.frequency  SampleTime=Ts
  Step : Step  Time=0.5  SampleTime=Ts
  Switch : Switch  Criteria=u2 > Threshold  SaturateOnIntegerOverflow=off  InputSameDT=off
  f : Outport
  wires:
  f_in/1 -> Switch/1
  Constant/1 -> Switch/3
  Step/1 -> Switch/2
  Switch/1 -> f/1

== system BatteryStoragePVPlantGFM/Conventional Source/Variant Subsystem/Synchronous Machine/Governor and Prime Mover /Governor ==
  pu_velocity : Inport
  1/T_G : Gain  Gain=1/T_G
  1/droop : Gain  Gain=1/(droop_percentage/100)
  Delta load setpoint : Sum  Inputs=+-|
  Delta speed : Sum  Inputs=-+|
  Discrete-Time Integrator : DiscreteIntegrator  InitialCondition=pu_torque0  SampleTime=Ts  ICPrevOutput=DiscIntNeverNeededParam  ICPrevScaledInput=DiscIntNeverNeededParam
  Load_setpoint : Constant  Value=pu_load_reference_setpoint  SampleTime=Ts
  Speed_ref : Constant  Value=pu_speed_reference  SampleTime=Ts
  Subtract : Sum  Inputs=|+-
  delta_y : Outport  VectorParamsAs1DForOutWhenUnconnected=off
  wires:
  Speed_ref/1 -> Delta speed/1
  Delta speed/1 -> 1/droop/1
  Load_setpoint/1 -> Delta load setpoint/1
  pu_velocity/1 -> Delta speed/2
  1/droop/1 -> Delta load setpoint/2
  Delta load setpoint/1 -> Subtract/1
  Subtract/1 -> 1/T_G/1
  1/T_G/1 -> Discrete-Time Integrator/1
  Discrete-Time Integrator/1 -> delta_y/1, Subtract/2

== system BatteryStoragePVPlantGFM/Conventional Source/Variant Subsystem/Synchronous Machine/Governor and Prime Mover /Non-reheat turbine ==
  delta_y : Inport
  1/T_CH : Gain  Gain=1/T_CH
  Discrete-Time Integrator : DiscreteIntegrator  InitialCondition=pu_torque0  SampleTime=Ts  ICPrevOutput=DiscIntNeverNeededParam  ICPrevScaledInput=DiscIntNeverNeededParam
  Sum : Sum  Inputs=|+-
  torque : Outport  VectorParamsAs1DForOutWhenUnconnected=off
  wires:
  delta_y/1 -> Sum/1
  Sum/1 -> 1/T_CH/1
  1/T_CH/1 -> Discrete-Time Integrator/1
  Discrete-Time Integrator/1 -> Sum/2, torque/1

== system BatteryStoragePVPlantGFM/BESS & PV PARK/100 MWp PV Park/PV Inverter A1/PV Controller/DC voltage controller & current reference/Current limits ==
  Imax : Inport
  iqref : Inport  Port=2
  idref : Inport  Port=3
  Constant8 : Constant  Value=0
  Constant9 : Constant  Value=0
  Sqrt : Sqrt
  Sqrt1 : Sqrt
  Square{1..4} (4 alike) : Math  Operator=square
  Step2 : Step  Time=0.01  SampleTime=Ts
  Step3 : Step  Time=0.01  SampleTime=Ts
  Sum6 : Sum  Inputs=|+-
  Sum9 : Sum  Inputs=|+-
  Switch1 : Switch  Threshold=.01  SaturateOnIntegerOverflow=off  InputSameDT=off
  Switch2 : Switch  Threshold=.01  SaturateOnIntegerOverflow=off  InputSameDT=off
  iubd : Outport
  iubq : Outport  Port=2
  wires:
  Sum9/1 -> Switch2/1
  Step3/1 -> Switch2/2
  Step2/1 -> Switch1/2
  Switch2/1 -> Sqrt1/1
  Square1/1 -> Sum6/1
  Switch1/1 -> Sqrt/1
  iqref/1 -> Square2/1
  Square3/1 -> Sum9/1
  Sum6/1 -> Switch1/1
  Square2/1 -> Sum6/2
  Constant8/1 -> Switch1/3
  Square4/1 -> Sum9/2
  Constant9/1 -> Switch2/3
  Sqrt/1 -> iubd/1
  Imax/1 -> Square3/1, Square1/1
  Sqrt1/1 -> iubq/1
  idref/1 -> Square4/1

== system BatteryStoragePVPlantGFM/BESS & PV PARK/100 MWp PV Park/PV Inverter A1/PV Controller/DC voltage controller & current reference/Subsystem ==
  V_mag : Inport
  iq_ub : Inport  Port=2
  LVRT.iq : Inport  Port=3
  Q_ref : Inport  Port=4
  Divide2 : Product  Inputs=*/
  Gain3 : Gain  Gain=-1
  Saturation Dynamic2 : simulink/Discontinuities/Saturation Dynamic  OutMin=[]  OutMax=[]  OutDataTypeStr=Inherit: Same as second input  OutDataType=fixdt(1, 16)  OutScaling=2^-10  DoSatur=off
  Switch6 : Switch  Threshold=.9  SaturateOnIntegerOverflow=off  InputSameDT=off
  iq_ub1 : InportShadow  Port=2
  Out1 : Outport
  wires:
  V_mag/1 -> Switch6/2, Divide2/2
  iq_ub1/1 -> Gain3/1
  Divide2/1 -> Saturation Dynamic2/2
  Q_ref/1 -> Divide2/1
  Gain3/1 -> Saturation Dynamic2/3
  iq_ub/1 -> Saturation Dynamic2/1
  Saturation Dynamic2/1 -> Switch6/1
  Switch6/1 -> Out1/1
  LVRT.iq/1 -> Switch6/3

== system BatteryStoragePVPlantGFM/BESS & PV PARK/100 MWp PV Park/PV Inverter A1/PV Controller/DC voltage controller & current reference/Subsystem1 ==
  Vmag : Inport
  P_pv : Inport  Port=2
  PV_Mpp_vdc : Inport  Port=3
  PV_vdc : Inport  Port=4
  id_ub : Inport  Port=5
  Constant4 : Constant  Value=0
  Divide : Product  Inputs=/*
  Gain4 : Gain  Gain=1/(1*Base.MVA_base_new)
  Saturation Dynamic1 : simulink/Discontinuities/Saturation Dynamic  OutMin=[]  OutMax=[]  OutDataTypeStr=Inherit: Same as second input  OutDataType=fixdt(1, 16)  OutScaling=2^-10  DoSatur=off
  Sum : Sum  Inputs=|++
  V_dc_Controller1 : Subsystem
  Out1 : Outport
  wires:
  Constant4/1 -> Saturation Dynamic1/3
  P_pv/1 -> Gain4/1
  V_dc_Controller1/1(Out1) -> Sum/2
  Sum/1 -> Saturation Dynamic1/2
  Vmag/1 -> Divide/1
  PV_vdc/1 -> V_dc_Controller1/2(In2)
  id_ub/1 -> Saturation Dynamic1/1
  Gain4/1 -> Divide/2
  Divide/1 -> Sum/1
  Saturation Dynamic1/1 -> Out1/1
  PV_Mpp_vdc/1 -> V_dc_Controller1/1(PV_plant1)

== system BatteryStoragePVPlantGFM/BESS & PV PARK/100 MWp PV Park/PV Inverter A2/PV Controller/DC voltage controller & current reference/Current limits ==
  Imax : Inport
  iqref : Inport  Port=2
  idref : Inport  Port=3
  Constant8 : Constant  Value=0
  Constant9 : Constant  Value=0
  Sqrt : Sqrt
  Sqrt1 : Sqrt
  Square{1..4} (4 alike) : Math  Operator=square
  Step2 : Step  Time=0.01  SampleTime=Ts
  Step3 : Step  Time=0.01  SampleTime=Ts
  Sum6 : Sum  Inputs=|+-
  Sum9 : Sum  Inputs=|+-
  Switch1 : Switch  Threshold=.01  SaturateOnIntegerOverflow=off  InputSameDT=off
  Switch2 : Switch  Threshold=.01  SaturateOnIntegerOverflow=off  InputSameDT=off
  iubd : Outport
  iubq : Outport  Port=2
  wires:
  Sum9/1 -> Switch2/1
  Step3/1 -> Switch2/2
  Step2/1 -> Switch1/2
  Switch2/1 -> Sqrt1/1
  Square1/1 -> Sum6/1
  Switch1/1 -> Sqrt/1
  iqref/1 -> Square2/1
  Square3/1 -> Sum9/1
  Sum6/1 -> Switch1/1
  Square2/1 -> Sum6/2
  Constant8/1 -> Switch1/3
  Square4/1 -> Sum9/2
  Constant9/1 -> Switch2/3
  Sqrt/1 -> iubd/1
  Imax/1 -> Square3/1, Square1/1
  Sqrt1/1 -> iubq/1
  idref/1 -> Square4/1

== system BatteryStoragePVPlantGFM/BESS & PV PARK/100 MWp PV Park/PV Inverter A2/PV Controller/DC voltage controller & current reference/Subsystem ==
  V_mag : Inport
  iq_ub : Inport  Port=2
  LVRT.iq : Inport  Port=3
  Q_ref : Inport  Port=4
  Divide2 : Product  Inputs=*/
  Gain3 : Gain  Gain=-1
  Saturation Dynamic2 : simulink/Discontinuities/Saturation Dynamic  OutMin=[]  OutMax=[]  OutDataTypeStr=Inherit: Same as second input  OutDataType=fixdt(1, 16)  OutScaling=2^-10  DoSatur=off
  Switch6 : Switch  Threshold=.9  SaturateOnIntegerOverflow=off  InputSameDT=off
  iq_ub1 : InportShadow  Port=2
  Out1 : Outport
  wires:
  V_mag/1 -> Switch6/2, Divide2/2
  iq_ub1/1 -> Gain3/1
  Divide2/1 -> Saturation Dynamic2/2
  Q_ref/1 -> Divide2/1
  Gain3/1 -> Saturation Dynamic2/3
  iq_ub/1 -> Saturation Dynamic2/1
  Saturation Dynamic2/1 -> Switch6/1
  Switch6/1 -> Out1/1
  LVRT.iq/1 -> Switch6/3

== system BatteryStoragePVPlantGFM/BESS & PV PARK/100 MWp PV Park/PV Inverter A2/PV Controller/DC voltage controller & current reference/Subsystem1 ==
  Vmag : Inport
  P_pv : Inport  Port=2
  PV_Mpp_vdc : Inport  Port=3
  PV_vdc : Inport  Port=4
  id_ub : Inport  Port=5
  Constant4 : Constant  Value=0
  Divide : Product  Inputs=/*
  Gain4 : Gain  Gain=1/(1*Base.MVA_base_new)
  Saturation Dynamic1 : simulink/Discontinuities/Saturation Dynamic  OutMin=[]  OutMax=[]  OutDataTypeStr=Inherit: Same as second input  OutDataType=fixdt(1, 16)  OutScaling=2^-10  DoSatur=off
  Sum : Sum  Inputs=|++
  V_dc_Controller1 : Subsystem
  Out1 : Outport
  wires:
  Constant4/1 -> Saturation Dynamic1/3
  P_pv/1 -> Gain4/1
  V_dc_Controller1/1(Out1) -> Sum/2
  Sum/1 -> Saturation Dynamic1/2
  Vmag/1 -> Divide/1
  PV_vdc/1 -> V_dc_Controller1/2(In2)
  id_ub/1 -> Saturation Dynamic1/1
  Gain4/1 -> Divide/2
  Divide/1 -> Sum/1
  Saturation Dynamic1/1 -> Out1/1
  PV_Mpp_vdc/1 -> V_dc_Controller1/1(PV_plant1)
